simulink model "light_test"  (R2019b)
settings: Solver=FixedStepAuto  StartTime=0.0  StopTime=inf  FixedStep=0.001  RelTol=1e-3
undefined symbols (not defined in the file or in its folder): Standard_Devices, UDP_Protocol
libraries: simulink x4, simulink_extras x3, sldrtlib x3
settings Model: Creator=guy-m  LastModifiedBy=guy-m
settings RTWCC: Description=Simulink Desktop Real-Time  SystemTargetFile=sldrt.tlc  TemplateMakefile=sldrt.tmf  RTWCompilerOptimization=on
settings CodeAppCC: MaxIdLength=95
settings SimulinkDesktopRealTimeCC: TargetPreCompLibLocation=C:\Program Files\MATLAB\R2019b\toolbox\sldrt\lib\win64  PreserveStateflowLocalDataDimensions=off

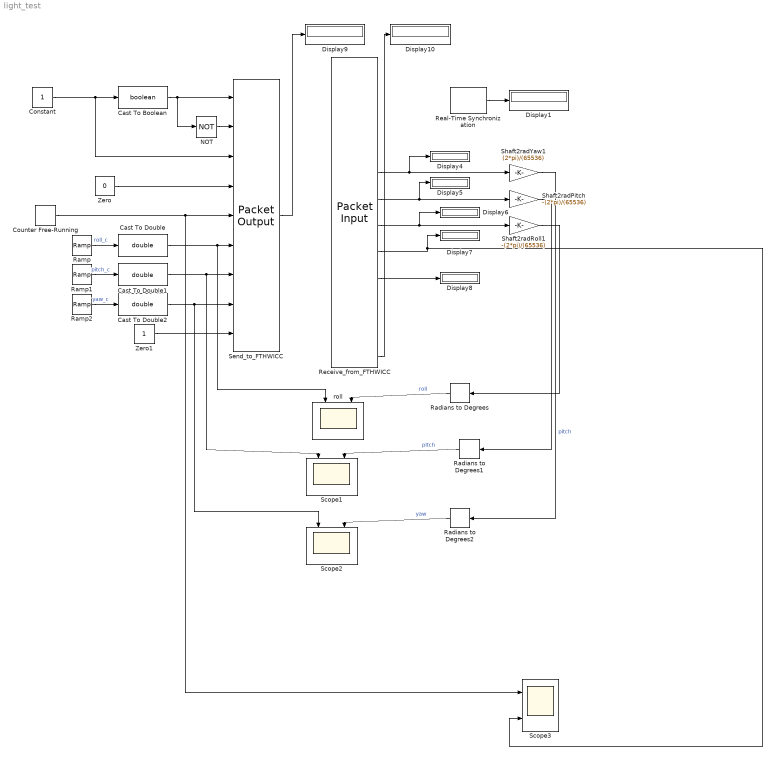
== system light_test ==
  Cast To Boolean : DataTypeConversion  OutDataTypeStr=boolean
  Cast To Double : DataTypeConversion  OutDataTypeStr=double
  Cast To Double1 : DataTypeConversion  OutDataTypeStr=double
  Cast To Double2 : DataTypeConversion  OutDataTypeStr=double
  Constant : Constant
  Counter Free-Running : simulink/Sources/Counter Free-Running  NumBits=16  tsamp=-1
  Display{1,4..10} (8 alike) : Display
  NOT : Logic  Operator=NOT  IconShape=distinctive  AllPortsSameDT=off  OutDataTypeStr=boolean
  Radians to Degrees : simulink_extras/Transformations/Radians to Degrees
  Radians to Degrees1 : simulink_extras/Transformations/Radians to Degrees
  Radians to Degrees2 : simulink_extras/Transformations/Radians to Degrees
  Ramp : simulink/Sources/Ramp  slope=45  start=0  InitialOutput=0
  Ramp1 : simulink/Sources/Ramp  slope=0  start=0  InitialOutput=0
  Ramp2 : simulink/Sources/Ramp  slope=0  start=0  InitialOutput=0
  Real-Time Synchronization : sldrtlib/Real-Time Synchronization  SampleTime=1/100  MaxMissedTicks=100  ShowMissedTicks=on  YieldWhenWaiting=off
  Receive_from_FTHWICC : sldrtlib/Packet Input  SampleTime=1/100  MaxMissedTicks=1000  ShowMissedTicks=on  YieldWhenWaiting=on  DrvName=Standard_Devices/UDP_Protocol  DrvAddress=36864  DrvOptions=[0 36880 49 57 50 46 49 54 56 46 49 46 49 53 54 0 0 0 0 0 0 0 0 0 0 0 0 0 0 0 0 0 0 0 0 0 0 0 0 0 0 0 0 0 0 0 0 0 0 0 0 0 0 0 0 0 0 0 0 0 0 0 0 0 0 0 0 0 0 0 0 0 0 0 0 0 0 0 0 0 0 0 0 0 0 0 0 0 0 0 0 0 0 0 0 0 0 0 0 0 0 0 0 0 0 0 0 0 0 0 0 0 0 0 0 0 0 0 0 0 0 0 0 0 0 0 0 0 0 0 0 0 0 0 0 0 0 0 0 0 0 0 0 0 0 0 0 0 0 0 0 0 0 0 0 0 0 0 0 0 0 0 0 0 0 0 0 0 0 0 0 0 0 0 0 0 0 0 0 0 0 0 0 0 0 0 0 0 0 0 0 0 0 0 0 0 0 0 0 0 0 0 0 0 0 0 0 0 0 0 0 0 0 0 0 0 0 0 0 0 0 0 0 0 0 0 0 0 0 0 0 0 0 0 0 0 0 0 0 0 0 0 0 0 0 0 0 0 0 0 0 0 0 0 0 0]  PacketSize=66  DataTypes={'double','double','double','double','double','double','double','uint16','double'}  ShowReady=on  ShowError=on  PacketID=1  ByteOrder=1  ShowTimestamp=off
      settings: AttributesFormatString=UDP Protocol [36864]  SourceProductName=Simulink Desktop Real-Time
  Scope1 : Scope  NumInputPorts=2
  Scope2 : Scope  NumInputPorts=2
  Scope3 : Scope  NumInputPorts=2
  Send_to_FTHWICC : sldrtlib/Packet Output  SampleTime=1/100  MaxMissedTicks=1000  ShowMissedTicks=on  YieldWhenWaiting=on  DrvName=Standard_Devices/UDP_Protocol  DrvAddress=36864  DrvOptions=[0 36880 49 57 50 46 49 54 56 46 49 46 49 53 54 0 0 0 0 0 0 0 0 0 0 0 0 0 0 0 0 0 0 0 0 0 0 0 0 0 0 0 0 0 0 0 0 0 0 0 0 0 0 0 0 0 0 0 0 0 0 0 0 0 0 0 0 0 0 0 0 0 0 0 0 0 0 0 0 0 0 0 0 0 0 0 0 0 0 0 0 0 0 0 0 0 0 0 0 0 0 0 0 0 0 0 0 0 0 0 0 0 0 0 0 0 0 0 0 0 0 0 0 0 0 0 0 0 0 0 0 0 0 0 0 0 0 0 0 0 0 0 0 0 0 0 0 0 0 0 0 0 0 0 0 0 0 0 0 0 0 0 0 0 0 0 0 0 0 0 0 0 0 0 0 0 0 0 0 0 0 0 0 0 0 0 0 0 0 0 0 0 0 0 0 0 0 0 0 0 0 0 0 0 0 0 0 0 0 0 0 0 0 0 0 0 0 0 0 0 0 0 0 0 0 0 0 0 0 0 0 0 0 0 0 0 0 0 0 0 0 0 0 0 0 0 0 0 0 0 0 0 0 0 0 0]  PacketSize=52  DataTypes={'boolean','boolean','double','double','uint16','double','double','double','double'}  ShowReady=off  ShowError=off  PacketID=1  ByteOrder=1  InitialValue=[]  FinalValue=[]
      settings: AttributesFormatString=UDP Protocol [36864]  SourceProductName=Simulink Desktop Real-Time
  Shaft2radPitch : Gain  Gain=-(2*pi)/(65536)
  Shaft2radRoll1 : Gain  Gain=-(2*pi)/(65536)
  Shaft2radYaw1 : Gain  Gain=(2*pi)/(65536)
  Zero : Constant  Value=0  OutDataTypeStr=Inherit: Inherit via back propagation
  Zero1 : Constant  OutDataTypeStr=Inherit: Inherit via back propagation
  roll : Scope  NumInputPorts=2
  wires:
  Constant/1 -> Send_to_FTHWICC/3, Cast To Boolean/1
  Cast To Boolean/1 -> NOT/1, Send_to_FTHWICC/1
  NOT/1 -> Send_to_FTHWICC/2
  Zero/1 -> Send_to_FTHWICC/4
  Counter Free-Running/1 -> Scope3/1, Send_to_FTHWICC/5
  Zero1/1 -> Send_to_FTHWICC/9
  Ramp/1 -> Cast To Double/1  "roll_c"
  Ramp2/1 -> Cast To Double2/1  "yaw_c"
  ? -> ?
  Receive_from_FTHWICC/6 -> Shaft2radPitch/1, Display5/1
  Receive_from_FTHWICC/5 -> Shaft2radYaw1/1, Display4/1
  Receive_from_FTHWICC/9 -> Display8/1
  Receive_from_FTHWICC/7 -> Shaft2radRoll1/1, Display6/1
  Ramp1/1 -> Cast To Double1/1  "pitch_c"
  Receive_from_FTHWICC/8 -> Scope3/2, Display7/1
  Send_to_FTHWICC/1 -> Display9/1
  Receive_from_FTHWICC/12 -> Display10/1
  Shaft2radRoll1/1 -> Radians to Degrees/1
  Radians to Degrees/1 -> roll/2  "roll"
  Radians to Degrees1/1 -> Scope1/2  "pitch"
  Radians to Degrees2/1 -> Scope2/2  "yaw"
  Shaft2radPitch/1 -> Radians to Degrees1/1
  Shaft2radYaw1/1 -> Radians to Degrees2/1  "pitch"
  Real-Time Synchronization/1 -> Display1/1
  Cast To Double/1 -> roll/1, Send_to_FTHWICC/6
  Cast To Double1/1 -> Send_to_FTHWICC/7, Scope1/1
  Cast To Double2/1 -> Scope2/1, Send_to_FTHWICC/8
